simulink model "Lunar_Rocker_N_Arm95_unity"  (R2023b)
settings: Solver=VariableStepAuto  StartTime=0.0  StopTime=160  RelTol=1e-3
libraries: dspnetwork x8, sldrtlib x1
settings Model: Creator=dr  LastModifiedBy=jeric
settings DebuggingCC: UnconnectedInputMsg=warning  UnconnectedOutputMsg=warning  UnconnectedLineMsg=warning
settings ModelReferenceCC: EnableRefExpFcnMdlSchedulingChecks=on
settings RTWCC: DLArmComputeVersion=19.05

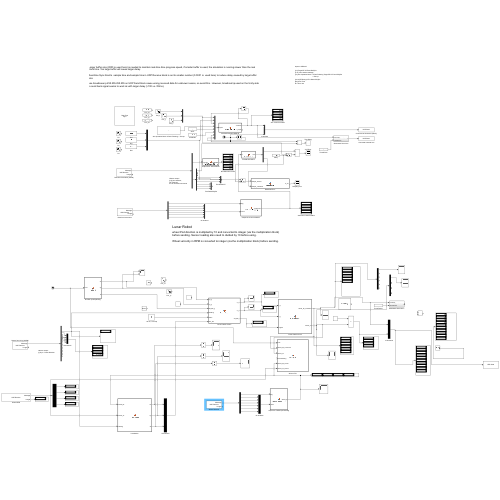
[thumbnail: Simulink's stored preview of the top-level diagram]
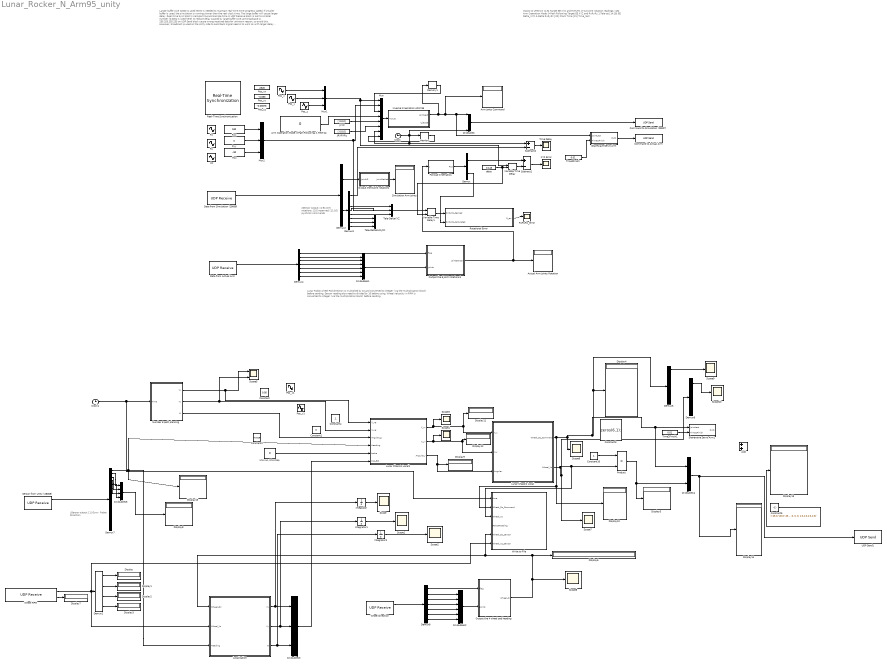
== system Lunar_Rocker_N_Arm95_unity ==
  note: //Sensor output:
      | [1:9] joint rotations;
      | [10] reserved;
      | [11:16] joysticks commands
  note: Larger buffer size {2000 is used here} is needed to maintain real-time time progress speed, if smaller buffer is used, the simulation is running slower than the real clock time. Too large buffer will cause larger delay.
      |
      | Real-time Sync block's sample time and sample time in UDP Receive block is set to smaller number (0.0001 is used here) to reduce delay caused by large buffer size
      |
      | use broadcase ip 255.255.255.255 on UDP Send block cause wrong received data for unknown reason, so avoid this. However, broadcast ip used on the Unity side to send back signal seems to work ok with larger delay (>100 vs <50ms).
  note: Inputs to UR3InvK
      |
      | [1:6] Target EE XYZ and RxRyRz
      | [7:12] Joint rotation readings;
      | [13] Arm Operation Mode: 	0-Path Following Target EE XYZ and RxRyRz
      | 						1:Tele-op
      |
      | [14:19] EE Delta_XYZ & Delta RxRyRz
      | [20] Clock Time
      | [21] Time_last
  note: //Sensor output:
      | [1] Gyro - Robot Direction
  note: Lunar Robot
      |
      | wheel Pod direction is multiplied by 10 and converted to integer (via the multiplication block) before sending. Sensor reading also need to divided by 10 before using.
      |
      | Wheel velcocity in RPM is converted to integer (via the multiplication block) before sending.
  "1 to run, 0 to stop" : Constant  Value=0  OutDataTypeStr=double  SampleTime=0.01
  10 doubles : Mux  Inputs=5
  10 doubles1 : Mux  Inputs=6
  10 doubles2 : Mux  Inputs=6
  10 doubles3 : Mux  Inputs=3
  10 doubles4 : Mux  Inputs=2
  10 doubles5 : Mux
  Actual Arm Joints Rotation : Display
      settings: Decimation=4
  Add : Sum
  Arm Jonts Command : Display
      settings: Decimation=4
  Arm Operation Mode: 0 Path Following; 1 Tele-op : Constant  Value=0
  Clock : Clock
  Clock1 : Clock
  Command to Actual Arm : dspnetwork/UDP Send  remoteURL='192.168.0.226'  remotePort=20001  localURL='0.0.0.0'  localPortSource=Automatically determine  localPort=-1  sendBufferSize=8192  sampletime=-1  blockPlatform=[]  separateLengthPort=0
  Command to Simulation (29007) : dspnetwork/UDP Send  remoteURL='127.0.0.1'  remotePort=29007  localURL='0.0.0.0'  localPortSource=Automatically determine  localPort=-1  sendBufferSize=2500  sampletime=-1  blockPlatform=[]  separateLengthPort=0
  Constant : Constant  Value=0.05  OutDataTypeStr=double  SampleTime=0.1
  Constant1 : Constant  Value=0  OutDataTypeStr=double  SampleTime=0.1
  Constant10 : Constant  OutDataTypeStr=int16
  Constant2 : Constant  Value=-0.628  OutDataTypeStr=double  SampleTime=0.01
  Constant3 : Constant  Value=zeros(6,1);  OutDataTypeStr=int16
  Constant4 : Constant  Value=.1  OutDataTypeStr=double  SampleTime=0.1
  Constant5 : Constant  Value=[-45.0,-45.0,-45.0,-45.0, 0, 0, 1.0,1.0,1.0,1.0]'  OutDataTypeStr=double  SampleTime=0.1
  Data from Actual Arm : dspnetwork/UDP Receive  localURL='0.0.0.0'  localPort=20001  remoteURL='0.0.0.0'  remotePort=-1  recvBufferSize=8192  dims=7  signalDatatype=int16  isComplex=off  isVarSize=off  showBlockingTime=off  blockingTime=0  sampletime=0.0001  blockPlatform=[]
  Data from Simulation (29008) : dspnetwork/UDP Receive  localURL='0.0.0.0'  localPort=29008  remoteURL='127.0.0.1'  remotePort=-1  recvBufferSize=2500  dims=18  signalDatatype=double  isComplex=off  isVarSize=off  showBlockingTime=off  blockingTime=0  sampletime=0.0001  blockPlatform=[]
  Demux : Demux  Outputs=2
  Demux1 : Demux
  Demux2 : Demux  Outputs=2
  Demux3 : Demux  Outputs=9
  Demux4 : Demux  Outputs=7
  Demux5 : Demux  Outputs=6
  Demux6 : Demux
  Demux7 : Demux  Outputs=18
  Demux8 : Demux  Outputs=7
  Display{,1..15} (16 alike) : Display
      Display10 settings: Decimation=4
      Display11 settings: Decimation=4
      Display12 settings: Decimation=4
      Display13 settings: Decimation=4
      Display14 settings: Decimation=4
      Display15 settings: Decimation=4
      Display4 settings: Decimation=6
      Display5 settings: Decimation=4
      Display8 settings: Decimation=4
      Display9 settings: Decimation=4
  Forwad Kinematics : MATLAB Function  TreatAsAtomicUnit=on
  Integrator : Integrator
  Integrator1 : Integrator
  Integrator2 : Integrator
  Inverse Kinematics ARM 95 : MATLAB Function  TreatAsAtomicUnit=on  SystemSampleTime=0.01
  JRXRYRz : Constant  Value=[ 0,0,0]
  JXYZ : Constant  Value=[ 0,0,0]
  Localization : MATLAB Function  TreatAsAtomicUnit=on
  Lunar Chassis Local : MATLAB Function  TreatAsAtomicUnit=on
  Lunar Chassis Local1 : MATLAB Function  TreatAsAtomicUnit=on
  Memory : Memory  InheritSampleTime=on
  Memory1 : Memory  InitialCondition=[0,45,-75,120,90,0]'  InheritSampleTime=on  LinearizeMemory=on  LinearizeAsDelay=on
  Mux : Mux  Inputs=8
  Mux1 : Mux  Inputs=3
  Mux2 : Mux  Inputs=3
  Number 8 path planning : MATLAB Function  TreatAsAtomicUnit=on
  Output the 4 wheel pod heading : MATLAB Function  TreatAsAtomicUnit=on
  Output the 6 Joint rotations : MATLAB Function  TreatAsAtomicUnit=on
  Output the 6 Joint rotations1 : MATLAB Function  TreatAsAtomicUnit=on
  Pos_x : Sin  Amplitude=0.075  Bias=.2595  Frequency=1.57  Phase=1.57  SampleTime=0.01
  Pos_x1 : Sin  Amplitude=.05  Frequency=0.157  SampleTime=0.01
  Pos_xx : Constant  Value=.2345
  Pos_y : Sin  Amplitude=0.15  Bias=-0.053  Frequency=1.57  SampleTime=0.01
  Pos_y1 : Sin  Amplitude=.05  Frequency=0.157  Phase=1.57  SampleTime=0.01
  Pos_yy : Constant  Value=-0.053
  Pos_z : Sin  Amplitude=0.03  Bias=-0.03676  Frequency=6.28  SampleTime=0.01
  Pos_zz : Constant  Value=-0.03676
  Product : Product  OutDataTypeStr=double
  Real-Time Synchronization : sldrtlib/Real-Time Synchronization  SampleTime=0.01  MaxMissedTicks=10000000  ShowMissedTicks=off  YieldWhenWaiting=on
  Rotational Error : MATLAB Function  TreatAsAtomicUnit=on
  Rx : Sin  Amplitude=45  Frequency=.628  SampleTime=0.01
  RxRyRz_Error : Scope
  Rxx : Constant  Value=180
  Ry : Sin  Amplitude=45  Frequency=0.785  SampleTime=0.01
  Ryy : Constant  Value=0
  Rz : Sin  Amplitude=90  Bias=-90  Frequency=0.785  SampleTime=0.01
  Rzz : Constant  Value=-90
  Scope{,1..4,6..10} (10 alike) : Scope
  Scope5 : Scope  NumInputPorts=2
  Sensor from Unity (28008) : dspnetwork/UDP Receive  localURL='0.0.0.0'  localPort=28008  remoteURL='127.0.0.1'  remotePort=-1  recvBufferSize=2500  dims=18  signalDatatype=double  isComplex=off  isVarSize=off  showBlockingTime=off  blockingTime=0  sampletime=0.0001  blockPlatform=[]
  Sharewave Servo Arm : Subsystem
  Sharewave Servo Arm1 : Subsystem
  Simulation Arm Joints : Display
      settings: Decimation=4
  Subtract1 : Sum  Inputs=+-
  Subtract2 : Sum  Inputs=+-
  Tele-DeltaRxRyRz : Mux  Inputs=3
  Tele-DeltaXYZ : Mux  Inputs=3
  Time Delay : Scope
  Time2Finish : Constant  Value=0.01
  Time2Finish1 : Constant  Value=0.01
  UDP Send1 : dspnetwork/UDP Send  remoteURL='127.0.0.1'  remotePort=28007  localURL='0.0.0.0'  localPortSource=Automatically determine  localPort=-1  sendBufferSize=8192  sampletime=-1  blockPlatform=[]  separateLengthPort=0
  Variable Time Delay : VariableTransportDelay  MaximumDelay=10  ZeroDelay=on
  Variable Time Delay1 : VariableTransportDelay  MaximumDelay=10  ZeroDelay=on
  Wheel Direction : dspnetwork/UDP Receive  localURL='0.0.0.0'  localPort=20004  remoteURL='0.0.0.0'  remotePort=-1  recvBufferSize=8192  dims=7  signalDatatype=int16  isComplex=off  isVarSize=off  showBlockingTime=off  blockingTime=0  sampletime=0.0001  blockPlatform=[]
  Wheel RPM : dspnetwork/UDP Receive  localURL='0.0.0.0'  localPort=20002  remoteURL='0.0.0.0'  remotePort=-1  recvBufferSize=8192  dims=4  signalDatatype=int16  isComplex=off  isVarSize=off  showBlockingTime=off  blockingTime=0  sampletime=0.0001  blockPlatform=[]
  Write to File : MATLAB Function  TreatAsAtomicUnit=on
  XYZ Error : Scope
  delay : Constant  Value=0.145
  wires:
  Mux/1 -> Inverse Kinematics ARM 95/1(Inputs)
  Data from Simulation (29008)/1 -> Demux2/1
  Inverse Kinematics ARM 95/1(JointLast) -> Arm Jonts Command/1, Sharewave Servo Arm/1(JointLast), 10 doubles/1, Memory1/1
  Demux/2 -> Rotational Error/2(RxRyRz_calculated)
  Demux/1 -> Subtract1/1
  Subtract1/1 -> XYZ Error/1
  Mux2/1 -> Variable Time Delay1/1, Mux/2
  Forwad Kinematics/1(Pos) -> Demux/1
  Clock/1 -> 10 doubles/5, Mux/7, Subtract2/1, Memory/1
  Memory/1 -> Mux/8
  Mux1/1 -> Variable Time Delay/1, Mux/1
  Demux2/2 -> Demux3/1
  Arm Operation Mode: 0 Path Following; 1 Tele-op/1 -> Mux/4
  Subtract2/1 -> Time Delay/1
  Demux3/1 -> Subtract2/2
  JXYZ/1 -> Mux/5
  JRXRYRz/1 -> Mux/6
  Rotational Error/1(R_err) -> RxRyRz_Error/1
  Sharewave Servo Arm/1(Out1) -> Command to Actual Arm/1
  Time2Finish/1 -> Sharewave Servo Arm/2(Time2Finish)
  Variable Time Delay/1 -> Subtract1/2
  Rxx/1 -> Mux2/1
  Ryy/1 -> Mux2/2
  Rzz/1 -> Mux2/3
  Demux4/4 -> 10 doubles1/3
  Output the 6 Joint rotations1/1(JointSensor) -> Forwad Kinematics/1(J), Actual Arm Joints Rotation/1
  Demux4/3 -> 10 doubles1/2
  Demux4/2 -> 10 doubles1/1
  10 doubles1/1 -> Output the 6 Joint rotations1/2(Joints)
  Demux4/6 -> 10 doubles1/5
  Demux4/1 -> Output the 6 Joint rotations1/1(flag)
  Data from Actual Arm/1 -> Demux4/1
  Demux4/7 -> 10 doubles1/6
  Demux4/5 -> 10 doubles1/4
  Memory1/1 -> Mux/3
  delay/1 -> Variable Time Delay1/2, Variable Time Delay/2
  Variable Time Delay1/1 -> Rotational Error/1(RxRyRz_desired)
  Pos_x/1 -> Mux1/1
  Pos_y/1 -> Mux1/2
  Pos_z/1 -> Mux1/3
  Demux2/1 -> Output the 6 Joint rotations/1(JointVR)
  Output the 6 Joint rotations/1(JointMatlab) -> Simulation Arm Joints/1
  Demux3/8 -> Tele-DeltaRxRyRz/2
  Demux3/9 -> Tele-DeltaRxRyRz/3
  Demux3/6 -> Tele-DeltaXYZ/3
  Demux3/5 -> Tele-DeltaXYZ/2
  Demux3/7 -> Tele-DeltaRxRyRz/1
  Demux3/4 -> Tele-DeltaXYZ/1
  Demux8/5 -> 10 doubles2/4
  Number 8 path planning/2(Vy) -> Lunar Chassis Local1/2(V_yg), Scope5/2
  10 doubles4/1 -> UDP Send1/1, Display14/1
  Wheel RPM/1 -> Localization/2(Wheel_Vs), Write to File/6(Wheel_Vs_Sensor), Demux1/1
  Sensor from Unity (28008)/1 -> Demux7/1
  Lunar Chassis Local/2(Wheel_Vs) -> Write to File/3(Wheel_Vs), Product/2, Scope7/1, Demux6/1
  Demux8/6 -> 10 doubles2/5
  Demux1/3 -> Display2/1
  Demux1/4 -> Display3/1
  Localization/3(W) -> Integrator2/1, 10 doubles3/3
  Localization/2(Vy) -> Integrator1/1, 10 doubles3/2
  Integrator/1 -> Scope/1
  Constant5/1 -> Display13/1
  Demux6/1 -> Scope10/1
  Constant10/1 -> Product/1
  Demux8/2 -> 10 doubles2/1
  Lunar Chassis Local1/2(V_yr) -> Display12/1, Lunar Chassis Local/2(V_y), Scope4/1
  Wheel RPM/2 -> Display7/1
  Demux5/1 -> Scope9/1
  Integrator2/1 -> Scope2/1
  10 doubles5/1 -> Display8/1
  Demux7/2 -> 10 doubles5/1
  "1 to run, 0 to stop"/1 -> Lunar Chassis Local1/5(brake)
  Lunar Chassis Local/1(Wheel_Ds_Command) -> Display10/1, Write to File/2(Wheel_Ds_Command), 10 doubles4/1, Sharewave Servo Arm1/1(JointLast), Demux5/1, Display4/1, Scope6/1
  Output the 4 wheel pod heading/1(Wheel_D) -> Write to File/5(Wheel_Ds_sensor), Localization/1(Wheel_Ds), Display6/1, Scope8/1
  Demux7/3 -> 10 doubles5/2
  Demux8/7 -> 10 doubles2/6
  Demux7/1 -> Localization/3(Heading), Display15/1, Lunar Chassis Local1/4(Heading)
  Demux8/3 -> 10 doubles2/2
  Demux1/2 -> Display1/1
  10 doubles2/1 -> Output the 4 wheel pod heading/2(Joints)
  Demux8/4 -> 10 doubles2/3
  Lunar Chassis Local1/3(Angular_r) -> Display9/1, Lunar Chassis Local/3(Angular)
  Localization/1(Vx) -> Integrator/1, 10 doubles3/1
  Demux7/4 -> 10 doubles5/3
  Integrator1/1 -> Scope1/1
  Number 8 path planning/1(Vx) -> Lunar Chassis Local1/1(V_xg), Scope5/1
  Product/1 -> 10 doubles4/2, Display5/1
  Number 8 path planning/3(W) -> Lunar Chassis Local1/3(Angular_g)
  Demux8/1 -> Output the 4 wheel pod heading/1(flag)
  Lunar Chassis Local1/1(V_xr) -> Scope3/1, Display11/1, Lunar Chassis Local/1(V_x)
  Wheel Direction/1 -> Demux8/1
  Demux7/5 -> 10 doubles5/4
  10 doubles3/1 -> Lunar Chassis Local1/6(Pos_Est)
  Time2Finish1/1 -> Sharewave Servo Arm1/2(Time2Finish)
  Demux1/1 -> Display/1
  10 doubles/1 -> Command to Simulation (29007)/1
  Clock1/1 -> Write to File/1(time), Number 8 path planning/1(Time)

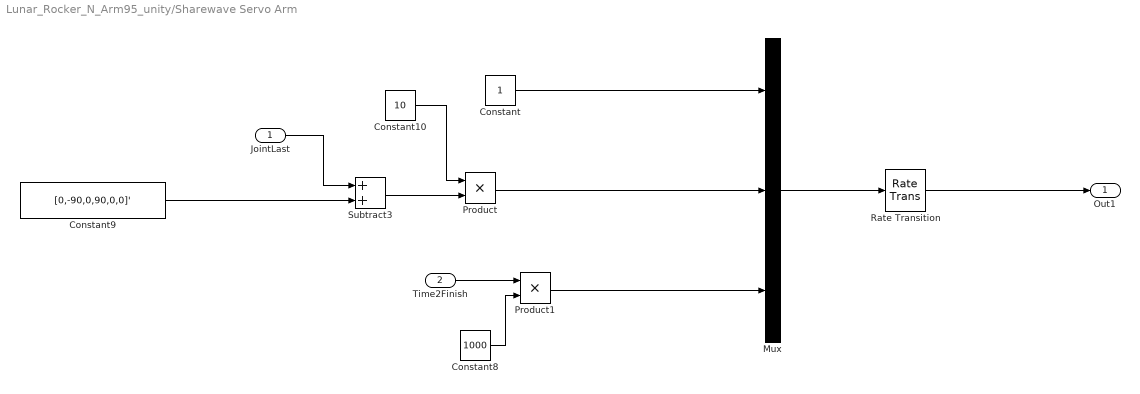
== system Lunar_Rocker_N_Arm95_unity/Sharewave Servo Arm ==
  JointLast : Inport
  Time2Finish : Inport  Port=2
  Constant : Constant  OutDataTypeStr=int16  SampleTime=0.1
  Constant10 : Constant  Value=10  OutDataTypeStr=int16
  Constant8 : Constant  Value=1000  OutDataTypeStr=int16
  Constant9 : Constant  Value=[0,-90,0,90,0,0]'  OutDataTypeStr=int16
  Mux : Mux  Inputs=3
  Product : Product  OutDataTypeStr=int16
  Product1 : Product  OutDataTypeStr=int16
  Rate Transition : RateTransition  OutPortSampleTime=0.01
  Subtract3 : Sum  OutDataTypeStr=int16
  Out1 : Outport
  wires:
  JointLast/1 -> Subtract3/1
  Mux/1 -> Rate Transition/1
  Constant/1 -> Mux/1
  Constant8/1 -> Product1/2
  Constant9/1 -> Subtract3/2
  Constant10/1 -> Product/1
  Subtract3/1 -> Product/2
  Rate Transition/1 -> Out1/1
  Product/1 -> Mux/2
  Time2Finish/1 -> Product1/1
  Product1/1 -> Mux/3

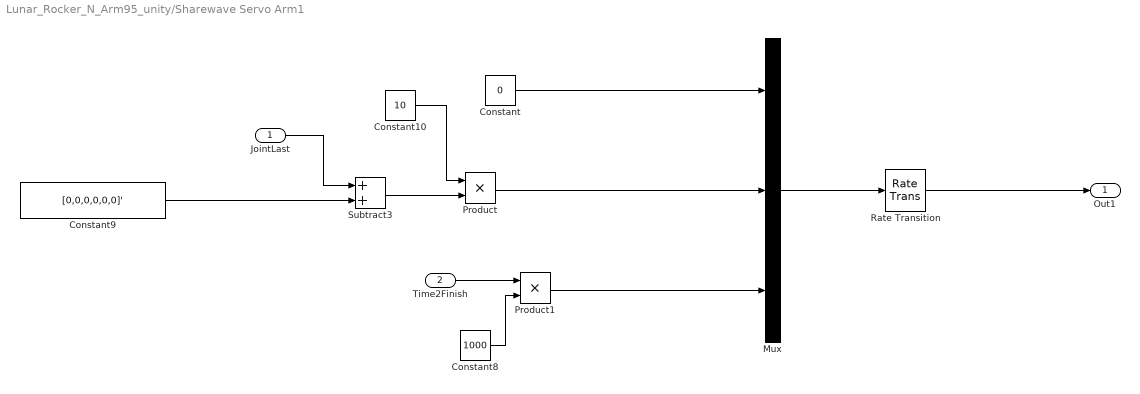
== system Lunar_Rocker_N_Arm95_unity/Sharewave Servo Arm1 ==
  JointLast : Inport
  Time2Finish : Inport  Port=2
  Constant : Constant  Value=0  OutDataTypeStr=int16  SampleTime=0.1
  Constant10 : Constant  Value=10  OutDataTypeStr=int16
  Constant8 : Constant  Value=1000  OutDataTypeStr=int16
  Constant9 : Constant  Value=[0,0,0,0,0,0]'  OutDataTypeStr=int16
  Mux : Mux  Inputs=3
  Product : Product  OutDataTypeStr=int16
  Product1 : Product  OutDataTypeStr=int16
  Rate Transition : RateTransition  OutPortSampleTime=0.01
  Subtract3 : Sum  OutDataTypeStr=int16
  Out1 : Outport
  wires:
  JointLast/1 -> Subtract3/1
  Mux/1 -> Rate Transition/1
  Constant/1 -> Mux/1
  Constant8/1 -> Product1/2
  Constant9/1 -> Subtract3/2
  Constant10/1 -> Product/1
  Subtract3/1 -> Product/2
  Rate Transition/1 -> Out1/1
  Product/1 -> Mux/2
  Time2Finish/1 -> Product1/1
  Product1/1 -> Mux/3

== matlab function Lunar_Rocker_N_Arm95_unity/Write to File ==
  settings: updateMethod=DISCRETE
  data: time input; Wheel_Ds_Command input; Wheel_Vs input; RobotHeading input; Wheel_Ds_sensor input; Wheel_Vs_Sensor input
function  WriteToFile(time, Wheel_Ds_Command, Wheel_Vs, RobotHeading, Wheel_Ds_sensor, Wheel_Vs_Sensor)
persistent  fileID; 

if isempty(fileID)
    fileID = fopen('log.txt','w');
    fprintf(fileID,'%6s %6s %6s %6s %6s %6s %6s %6s %6s','Time','D1','D2','D3','D4', 'V1','V2','V3','V4');
    fprintf(fileID,'%6s %6s %6s %6s %6s %6s %6s %6s %6s','Angle','D1_s','D2_s','D3_s','D4_s', 'V1_s','V2_s','V3_s','V4_s');
    fprintf(fileID,' \r\n');
end


fprintf(fileID,'%6.2f %6.1f %6.1f %6.1f %6.1f %6.1f %6.1f %6.1f %6.1f', time, Wheel_Ds_Command(1), Wheel_Ds_Command(2), Wheel_Ds_Command(3), Wheel_Ds_Command(4), Wheel_Vs(1), Wheel_Vs(2), Wheel_Vs(3), Wheel_Vs(4));
fprintf(fileID,'%6.1f %6.1f %6.1f %6.1f %6.1f %6d %6d %6d %6d', RobotHeading, Wheel_Ds_sensor(1), Wheel_Ds_sensor(2), Wheel_Ds_sensor(3), Wheel_Ds_sensor(4), Wheel_Vs_Sensor(1), Wheel_Vs_Sensor(2), Wheel_Vs_Sensor(3), Wheel_Vs_Sensor(4));
fprintf(fileID,' \r\n');

== matlab function Lunar_Rocker_N_Arm95_unity/Output the 6 Joint rotations ==
  data: JointVR input; JointMatlab output
function JointMatlab  = MatlabMaping6Joints(JointVR)
JointMatlab  = zeros (6,1);
JointMatlab(1:6) = JointVR(1:6);

== matlab function Lunar_Rocker_N_Arm95_unity/Forwad Kinematics ==
  data: J input; Pos output
function Pos  = LunarArmFK(J)
%UR3 robot arm

%cal Jacobian using 5.1.27, page 115, Robot Dyn and Control by Spong
Joint = zeros(6,1);
Pos = zeros(6,1);

Degree2Radian = pi/180;
 


%initial joint position
Joint(1)= J(1)*Degree2Radian;
Joint(2)= J(2)*Degree2Radian;
Joint(3)= J(3)*Degree2Radian;
Joint(4)= J(4)*Degree2Radian;
Joint(5)= J(5)*Degree2Radian;
Joint(6)= J(6)*Degree2Radian;
  

PTool=[0;0;0;1]; %The Tool or tip position expressed wrt the last frame physical dimension



dh = [   0              0           0           Joint(1); 
             pi/2           0           0           Joint(2);
             0              0.175       0           Joint(3);
             0              0.155        0.053           Joint(4);
             pi/2            0           0.0765     Joint(5);
             -pi/2           0           0.083     Joint(6)];

 
T=[1 0 0 0;0 1 0 0; 0 0 1 0; 0 0 0 1]; %INITIAL  Transformation matrix

for m=1:6
T=T*[cos(dh(m,4))                    -sin(dh(m,4))                0               dh(m,2)
    sin(dh(m,4))*cos(dh(m,1))   cos(dh(m,4))*cos(dh(m,1))   -sin(dh(m,1))       -sin(dh(m,1))*dh(m,3)
    sin(dh(m,4))*sin(dh(m,1))   cos(dh(m,4))*sin(dh(m,1))   cos(dh(m,1))       cos(dh(m,1))*dh(m,3)
    0                               0                           0               1];
%Axis(1:3,m)=T(1:3,3);
%Origin(1:3,m)= T(1:3,4);
end

PEndTemp=T*PTool;

Pos(1:3)= PEndTemp(1:3);
%[AXInitial,AYInitial,AZInitial] based on Fixed Angle
 

[Pos(4) Pos(5) Pos(6)]= R2FixAngle(T(1:3,1:3));
Pos(4:6) = Pos(4:6)/Degree2Radian;

function [AX,AY,AZ]= R2FixAngle(R) 

MINA=0.0001; %minimun we consider to be 0 degree

AY= atan2(-R(3,1), sqrt(R(1,1)^2+R(2,1)^2));

CAY=cos(AY);

if abs(CAY)>MINA
    AZ=atan2(R(2,1)/CAY, R(1,1)/CAY);
    AX=atan2(R(3,2)/CAY, R(3,3)/CAY);
elseif AY>0 % AY=90 degree
   AY=pi/2;
   AZ=0; %this is a convention to choose AZ to be zero, see page 47
   AX=atan2(R(1,2), R(2,2));
else  % AY=-90 degree
   AY=-pi/2;
   AZ=0; %this is a convention to choose AZ to be zero, see page 47
   AX=-atan2(R(1,2), R(2,2));
end

== matlab function Lunar_Rocker_N_Arm95_unity/Rotational Error ==
  data: RxRyRz_desired input; R_err output; RxRyRz_calculated input
function R_err  = RotationErr(RxRyRz_desired, RxRyRz_calculated)

R1 = zeros(3,3);
R2 = zeros(3,3);
Rerror = zeros(3,3);

Degree2Radian = pi/180;
 
R1= FixAngle2R(RxRyRz_desired*Degree2Radian);
R2= FixAngle2R(RxRyRz_calculated*Degree2Radian);




Rerror = R1*(R2');
R_err = 0.5*[Rerror(3,2)-Rerror(2,3); Rerror(1,3)-Rerror(3,1);Rerror(2,1)-Rerror(1,2)];


%Fixed Angle representation page 45, intro to robotics
%Definition: Describing the orientation of frame B is as follows:
%start  with the frame coincident with a known reference frame A. First
%rotate B about axis XA by an angle AngleX, then rotate about YA by an
%angle AngleY, and then rotate about ZA by an angle AngleZ.

function [R]= FixAngle2R(AngleXYZ) 

cX  = cos (AngleXYZ(1));
sX  =   sin(AngleXYZ(1));
cY  =   cos (AngleXYZ(2));
sY  =   sin(AngleXYZ(2));
cZ  =   cos (AngleXYZ(3));
sZ  =   sin(AngleXYZ(3));

R=[cZ*cY cZ*sY*sX-sZ*cX cZ*sY*cX+sZ*sX;
   sZ*cY sZ*sY*sX+cZ*cX sZ*sY*cX-cZ*sX;
   -sY  cY*sX   cY*cX];

== matlab function Lunar_Rocker_N_Arm95_unity/Inverse Kinematics ARM 95 ==
  data: Inputs input; JointLast output; t_lapse output
function [JointLast, t_lapse]  = LunarArmInvK (Inputs)
persistent  PositionLast  RotationLast;

if isempty(PositionLast)
    PositionLast =zeros(3,1);
end

if isempty(RotationLast)
    RotationLast =zeros(3,1);
end

 
t_lapse = Inputs(20)- Inputs(21);

if Inputs(20) > 0.0 % delay start to make sure sensor data from the VR robot has arrived, during delay, send out the initial joint position 
 
% LEFT  ARM
% This function will generate the joint angle set for each joint on left
% arm based on drawing a circle on XZ plane, radius is RD.
% there are many import parameters is based on physical arm dimensions.
% please contact Dr Robot Inc for further information.

% The demo code is just for 'demo' use.

%cal Jacobian using 5.1.27, page 115, Robot Dyn and Control by Spong
%JInit

steps=5; 

Joint = zeros(6,steps+1);
JointWS = zeros(6,2);
Origin = zeros(3,6);
Axis = zeros(3,6);
PEnd = zeros (3,steps);
Jaco = zeros (6,6);
PTarget = zeros(3, steps+1);
FATarget = zeros(3, steps+1);
ODelta = zeros(3,steps);
WJointLtd = zeros (6,6);
JointLast = zeros (6,1);
RTeleDelta = eye(3,3);
finalPos = zeros(3,1);
finalRxRyRz = zeros(3,1);
PTeleDelta = zeros (3,1);  
Degree2Radian = pi/180;
RxRyRzTeleDelta = zeros(3,1);
RJ5 = zeros(3,3);

%initial joint position
Joint(1,1)= Inputs(7)*Degree2Radian;
Joint(2,1)= Inputs(8)*Degree2Radian;
Joint(3,1)= Inputs(9)*Degree2Radian;
Joint(4,1)= Inputs(10)*Degree2Radian;
Joint(5,1)= Inputs(11)*Degree2Radian;
Joint(6,1)= Inputs(12)*Degree2Radian;

%########################physical dimensions #############################
%Joint limit in degrees
JointLtd=[  -360,   360;
             -360,   360;
            -360,   360;
            -360,   360;
            -360,   360;
            -9000,   9000];
JointLtdExRate = 50; %Joint ltd avoidance exp increase rate, if this rate is too small, e.g. 10 or 1, it may exceed the limit a bit; 
JointSB=20; % safe zone before reaching joint limit, joint limit avoidance scheme starts action when entering the safe zone. effect grows exponentially
%Convert the safe operation zone (with a boundary of JointSB before the
%limit) from degree into the RAD
for i=1:6
           JointWS(i,1)=(JointLtd(i,1)+JointSB)*Degree2Radian;
           JointWS(i,2)=(JointLtd(i,2)-JointSB)*Degree2Radian;
end
       
T=[1 0 0 0;0 1 0 0; 0 0 1 0; 0 0 0 1]; %INITIAL  Transformation matrix
PTool=[0;0;0;1]; %The Tool or tip position expressed wrt the last frame physical dimension
%Catisian space task weighting, i.e. position and orientation tracking task
%weight, smaller , less significant to track, i.e. by setting WEnd(4,4)
%smaller (e.g. 0.01 while others are 1), the rotation along RX axis will not be tracked precisely.
%!!!!!!!!!!!!!!!!!!!!CHANGE HERE

WEnd=[1 0 0 0 0 0;
    0 1 0 0 0 0;
    0 0 1 0 0 0;
    0 0 0 .01 0 0;
    0 0 0 0 .01 0;
    0 0 0 0 0 .01];           %0.01

%Joint space weighting matrix, larger number will reduce the joint motion,
%i.e. the unit WJoint(6,6)=100, while others are "1" then the joint 6 will
%move very little.
%!!!!!!!!!!!!!!!!!!!!CHANGE HERE
WJoint=[1 0 0 0 0 0;
        0 1 0 0 0 0;
        0 0 1 0 0 0;
        0 0 0 .1 0 0;
        0 0 0 0 .1 0;
        0 0 0 0 0 .1];

 
DF2= 0.05; %0.15; %.015; %Damping factor square, larger, slower tracking, bigger tracking error, but more robust to singularity 


for k = 1:steps

    dh = [   0              0           0           Joint(1,k); 
             pi/2           0           0           Joint(2,k);
             0              0.175       0           Joint(3,k);
             0              0.155       0.053           Joint(4,k);
             pi/2            0           0.0765     Joint(5,k);
             -pi/2           0           0.083     Joint(6,k)];
 
T=[1 0 0 0;0 1 0 0; 0 0 1 0; 0 0 0 1]; %INITIAL  Transformation matrix

for m=1:6
T=T*[cos(dh(m,4))                    -sin(dh(m,4))                0               dh(m,2)
    sin(dh(m,4))*cos(dh(m,1))   cos(dh(m,4))*cos(dh(m,1))   -sin(dh(m,1))       -sin(dh(m,1))*dh(m,3)
    sin(dh(m,4))*sin(dh(m,1))   cos(dh(m,4))*sin(dh(m,1))   cos(dh(m,1))       cos(dh(m,1))*dh(m,3)
    0                               0                           0               1];
Axis(1:3,m)=T(1:3,3);
Origin(1:3,m)= T(1:3,4);
%if m==5 % copy the second last joint, (before the hand) Rotation
%    RJ5 = T(1:3,1:3);
%end

end

PEndTemp=T*PTool;
PEnd(1:3,k)=PEndTemp(1:3); %tip position in origin frame

%Jacobian upper part , i.e. the linear velocity part
Jaco(1:3,1)= cross (Axis (1:3,1), (PEnd (1:3,k) - Origin(1:3,1)));
Jaco(1:3,2)= cross (Axis (1:3,2), (PEnd (1:3,k)- Origin(1:3,2)));
Jaco(1:3,3)= cross (Axis (1:3,3), (PEnd (1:3,k)- Origin(1:3,3)));
Jaco(1:3,4)= cross (Axis (1:3,4), (PEnd (1:3,k)- Origin(1:3,4)));
Jaco(1:3,5)= cross (Axis (1:3,5), (PEnd (1:3,k)- Origin(1:3,5)));
Jaco(1:3,6)= cross (Axis (1:3,6), (PEnd (1:3,k)- Origin(1:3,6)));

%Jacobian lower part , i.e. the angular velocity part
Jaco(4:6,1)= Axis (1:3,1);
Jaco(4:6,2)= Axis (1:3,2);
Jaco(4:6,3)= Axis (1:3,3);
Jaco(4:6,4)= Axis (1:3,4);
Jaco(4:6,5)= Axis (1:3,5);
Jaco(4:6,6)= Axis (1:3,6);

if k==1 %cal the initial posotition and orientation from the initial joint reading
%target position, should use the sensor reading to calculate the X,Y,Z and
%plan the end effector motion accordingly to avoid rapid movement at start

PInitial    = PEnd(1:3,1);
RInitial    = T(1:3,1:3);
    
%Initialize the tip motion Target 
PTarget(1, 1) = PInitial(1);
PTarget(2, 1) = PInitial(2);
PTarget(3, 1) = PInitial(3) ;

InitialRxRyRZ=R2FixAngle(RInitial);
 
FATarget(1:3,1) = InitialRxRyRZ; %using Fixed-Angle representation page 47, intro to robotics

% set the final target position and RxRyRz
    if Inputs(13) >=1 % 1: tele-operation on end-effector, using Mode switching Initial pos + delat pos as the final target 
        magPosCommand = norm(Inputs(14:16));
        magRotCommand = norm(Inputs(17:19)); 

     if magPosCommand < 0.2  %no motion needed
         PTeleDelta = zeros(3,1);
     else
         PTeleDelta =RInitial*Inputs(14:16)*t_lapse*0.1;
     end

     if magRotCommand < 0.2 %no rotation needed
        RTeleDelta = eye(3,3);
     else
        RxRyRzTeleDelta = Inputs(17:19)*t_lapse*0.5;
        RTeleDelta = FixAngle2R (RxRyRzTeleDelta(1:3));   
     end
        
        finalPos = PositionLast + PTeleDelta;
        finalRxRyRz=R2FixAngle(FixAngle2R(RotationLast*Degree2Radian)*RTeleDelta)*180/pi;
        %finalRxRyRz = Inputs (4:6);
     
    else % =0 path following
        finalPos = Inputs (1:3);
        finalRxRyRz = Inputs (4:6);
    end
end    


%linear planning 
PTarget(1, k+1) = PTarget(1,1) + (finalPos(1)-PTarget(1,1))/steps*k;
PTarget(2, k+1) = PTarget(2,1) + (finalPos(2)-PTarget(2,1))/steps*k ;
PTarget(3, k+1) = PTarget(3,1) + (finalPos(3)-PTarget(3,1))/steps*k;
%PTarget(3, k+1) = PTarget(3,1) - RD - RD*cos(pi+ 2*pi*k/steps);


%planning the orientation motion

FATarget(1,k+1)= finalRxRyRz(1)*Degree2Radian ; 
FATarget(2,k+1)= finalRxRyRz(2)*Degree2Radian ;
FATarget(3,k+1)= finalRxRyRz(3)*Degree2Radian ;

RTarget = FixAngle2R(FATarget(1:3,k+1));

%tip motion delta
PDelta= PTarget(1:3,k+1)-PEnd(1:3,k);
%Rotation error
Rerror = RTarget*(T(1:3,1:3)');
ODelta(1:3,k) = 0.5*[Rerror(3,2)-Rerror(2,3); Rerror(1,3)-Rerror(3,1);Rerror(2,1)-Rerror(1,2)];

%Least square pseudo inverse of J
JacoP=Jaco(1:6,1:6);
%Jw=transpose(JacoP)*inv(JacoP*transpose(JacoP)+ DF2*eye(6));


%Joint limit avoidance
for i=1:6
    if Joint(i,k)>JointWS(i,2)
        JointOver= Joint(i,k)-JointWS(i,2);
    elseif     Joint(i,k) <JointWS(i,1)
        JointOver= JointWS(i,1)-Joint(i,k) ;
    else
       JointOver=0;     
   end   
WJointLtd(i,i)=WJoint(i,i)*exp(JointLtdExRate*JointOver); %Augment the WJoint weighting matrix with the Joint Limit Avoidance, closer to the limit, the Weighting unit will increase exponentially, and leading to smaller velocity till stop, therefore avoiding exceeding the limit
end

Jw=inv(transpose(JacoP)*WEnd*JacoP+ DF2*(WJointLtd))*transpose(JacoP)*WEnd;

%conJ=cond(JacoP)
%Jw=inv(Jaco);
%inverse kinematic of delta joint motion 

JDelta= Jw*[PDelta;ODelta(1:3,k)]; 

%orientation only
%Jw=W1*transpose(Jaco(4:6,1:6))*inv(Jaco(4:6,1:6)*W1*transpose(Jaco(4:6,1:6)));
%JDelta= Jw*[ODelta];

%with error on joint trackin
%Joint(1:6,k+2)=Joint(1:6,k+1)+JDelta + dot (JDelta, [0.5*(rand-0.5);0.5*(rand-0.5);0.5*(rand-0.5);0.5*(rand-0.5);0.2*(rand-0.5);0.2*(rand-0.5)]);
%here is what the robot arm controller should do: drive the arm to the
%position we need:
Joint(1:6,k+1)=Joint(1:6,k)+JDelta; 
end


JointLast(1:6) = Joint(1:6,k+1)/Degree2Radian;
PositionLast =  finalPos; %storrage of last pos target command 
RotationLast = finalRxRyRz;

else
    %initial position
    JointLast = [0, 45,-75, 120, 90, 0]';
    PositionLast =[0.3345, -0.053,-0.03676]';
    RotationLast = [180,0,-90]';
end
 

function AxAyAZ= R2FixAngle(R) 

MINA=0.0001; %minimun we consider to be 0 degree

AY= atan2(-R(3,1), sqrt(R(1,1)^2+R(2,1)^2));

CAY=cos(AY);

if abs(CAY)>MINA
    AZ=atan2(R(2,1)/CAY, R(1,1)/CAY);
    AX=atan2(R(3,2)/CAY, R(3,3)/CAY);
elseif AY>0 % AY=90 degree
   AY=pi/2;
   AZ=0; %this is a convention to choose AZ to be zero, see page 47
   AX=atan2(R(1,2), R(2,2));
else  % AY=-90 degree
   AY=-pi/2;
   AZ=0; %this is a convention to choose AZ to be zero, see page 47
   AX=-atan2(R(1,2), R(2,2));
end
AxAyAZ = [AX AY AZ]';

%Fixed Angle representation page 45, intro to robotics
%Definition: Describing the orientation of frame B is as follows:
%start  with the frame coincident with a known reference frame A. First
%rotate B about axis XA by an angle AngleX, then rotate about YA by an
%angle AngleY, and then rotate about ZA by an angle AngleZ.

function [R]= FixAngle2R(AngleXYZ) 

cX  = cos (AngleXYZ(1));
sX  =   sin(AngleXYZ(1));
cY  =   cos (AngleXYZ(2));
sY  =   sin(AngleXYZ(2));
cZ  =   cos (AngleXYZ(3));
sZ  =   sin(AngleXYZ(3));

R=[cZ*cY cZ*sY*sX-sZ*cX cZ*sY*cX+sZ*sX;
   sZ*cY sZ*sY*sX+cZ*cX sZ*sY*cX-cZ*sX;
   -sY  cY*sX   cY*cX];

== matlab function Lunar_Rocker_N_Arm95_unity/Localization ==
  data: Wheel_Ds input; Vx output; Vy output; W output; Wheel_Vs input; Heading input
function [Vx, Vy, W]  = Localization(Wheel_Ds, Wheel_Vs, Heading)

 

V_xr =0;
V_yr=0;
W=0;
PIH = zeros (3,8);
V_wheel = zeros(8,1);
V_robot = zeros(3,1);
 
Wheel_Ds  = double (Wheel_Ds  *pi/180.0);
 
V2RPM = 60.0/ (3.1415926*0.1);  % convert from m/s to RPM
 
Wheel_Vs = double (Wheel_Vs) /V2RPM;

L2 = 0.358/2.0; % half the length
W2 = 0.372/2.0;

H = [   1,  0,    -L2;
        0,  1,    -W2;
        1,  0,    -L2;
        0,  1,    W2;
        1,  0,    L2;
        0,  1,    -W2;
        1,  0,    L2;
        0,  1,    W2;];

PIH = inv(H'*H)*H';

for i =1:4
    V_wheel(2*i-1,1) = -Wheel_Vs(i)*sin(Wheel_Ds(i));
    V_wheel(2*i,1) = Wheel_Vs(i)*cos(Wheel_Ds(i));
end
V_robot = PIH*V_wheel;

V_xr = V_robot(1);
V_yr = V_robot(2);
W = V_robot(3) *180/pi;

%mapping to global frame

Heading = Heading  * 3.14/180;

Vx= (cos (Heading) *V_xr - sin(Heading) *V_yr) ;
Vy= (sin (Heading) *V_xr + cos(Heading) *V_yr) ;

== matlab function Lunar_Rocker_N_Arm95_unity/Output the 6 Joint rotations1 ==
  data: flag input; JointSensor output; Joints input
function JointSensor  = JointSensorMapping(flag, Joints)
persistent  Joints_last;
JointSensor =zeros(6,1);

if isempty(Joints_last)
    Joints_last =zeros(6,1);
end

if (flag == 1) && isempty (Joints) ~= true
    Joints_last = double (Joints)/10 - [0,-90,0,90,0,0]';
end

JointSensor = Joints_last;

== matlab function Lunar_Rocker_N_Arm95_unity/Lunar Chassis Local ==
  settings: updateMethod=DISCRETE
  data: V_x input; V_y input; Wheel_Ds_Command output; Angular input; Wheel_Vs output
function [Wheel_Ds_Command, Wheel_Vs]  = LunarChassis(V_x, V_y , Angular)
%output Wheel velocity in RPM

persistent Wheel_Ds_last Wheel_Ds_NoLimit Wheel_Ds_NoLimit_last ;  

if  isempty (Wheel_Ds_last) 
     Wheel_Ds_last =zeros(6,1);
end
if  isempty (Wheel_Ds_NoLimit) 
     Wheel_Ds_NoLimit = zeros(6,1);
     Wheel_Ds_NoLimit_last = zeros(6,1);
end
if  isempty (Wheel_Ds_NoLimit_last)
     Wheel_Ds_NoLimit_last = zeros(6,1);
end

 


Wheel_Ds= zeros(6,1); % only use the first 4, but the protocol needs a lenght of 6
Wheel_Vs= zeros(4,1);

Radian2Degree = 180/pi;
V2RPM = 60.0/ (3.1415926*0.1);  % convert from m/s to RPM
Length = 0.33472;
Width = 0.35038;

A = V_x + Angular *Length/2;
B = V_x - Angular *Length/2;
C = V_y + Angular *Width/2;

D = V_y - Angular *Width/2;
%LF
Wheel_Vs(1) = sqrt(B*B + D*D)*V2RPM;
Wheel_Ds(1) = -atan2(B,D)*Radian2Degree;
%RF
Wheel_Vs(2) = sqrt(B*B + C*C)*V2RPM;
Wheel_Ds(2) = -atan2(B,C)*Radian2Degree;
%LR
Wheel_Vs(3) = sqrt(A*A + D*D)*V2RPM ;
Wheel_Ds(3) = -atan2(A,D)*Radian2Degree;
%RR
Wheel_Vs(4) = sqrt(A*A + C*C)*V2RPM ;
Wheel_Ds(4) = -atan2(A,C)*Radian2Degree;

% Atan2 will return pi - -pi and may jump from pi to -pi, we need to
% process it, if the turning is over 180, take the direction with less
% truning, make sure turning is always less than 180

for i = 1:4 
    deltaRotation = Wheel_Ds(i) - Wheel_Ds_last(i);
    if (deltaRotation < -180)
        deltaRotation =   deltaRotation + 360;
    end
    if (deltaRotation > 180)
        deltaRotation = deltaRotation - 360;
    end
   
    Wheel_Ds_NoLimit(i) = Wheel_Ds_NoLimit(i)+ deltaRotation;
    Wheel_Ds_last(i)  = Wheel_Ds(i);
end



% since we could reverse the motor power instead turn the motor pod, if the
% turning is over 90 degree, we could reverse the wheel direction.

Wheel_Ds_Command = Wheel_Ds_NoLimit;

for i = 1:4
    if  Wheel_Ds_Command(i) -Wheel_Ds_NoLimit_last(i) > 90  
        Wheel_Ds_Command(i)= Wheel_Ds_Command(i)-180;
        Wheel_Vs(i) = - Wheel_Vs(i) ;
    elseif  Wheel_Ds_Command(i) -Wheel_Ds_NoLimit_last(i) < -90 
        Wheel_Ds_Command(i)= Wheel_Ds_Command(i) + 180;
        Wheel_Vs(i) = - Wheel_Vs(i) ;
    end
    Wheel_Ds_NoLimit_last(i) = Wheel_Ds_Command(i);
end

== matlab function Lunar_Rocker_N_Arm95_unity/Lunar Chassis Local1 ==
  data: V_xg input; V_yg input; V_xr output; Angular_g input; V_yr output; Heading input; Angular_r output; brake input; Pos_Est input
function [V_xr, V_yr, Angular_r]  = GlobaltoLocal(V_xg, V_yg , Angular_g, Heading, brake, Pos_Est)
%mapping global command to robot local frame
Heading = Heading  * 3.14/180;

V_xr =0;
V_yr =0;

% 
% persistent err_x_last err_y_last err_x_int err_y_int
% 
% if isempty(err_y_last)
%     err_x_last =0;
%     err_y_last =0;
%     err_x_int =0;
%     err_y_int =0;
% end
% err_x =0;
% err_y =0;
% % Kp control
% kp = 0;
% kd = 0;
% ki = 0.1;
% 
% 
% err_x = V_xg-Pos_Est(1);
% err_y = V_yg-Pos_Est(2);
% 
% err_x_int = err_x_int + err_x*0.01
% err_y_int = err_y_int + err_y*0.01
% 
% V_xg = V_xg + ki*err_x_int % + kp *err_x + kd*(err_x - err_x_last);
% V_yg = V_yg + ki*err_y_int %+ kp *err_y + kd*(err_y - err_y_last);
% 
% err_x_last = err_x;
% err_y_last = err_y;

V_xr= (cos (Heading) *V_xg + sin(Heading) *V_yg)*brake;
V_yr= (-sin (Heading) *V_xg + cos(Heading) *V_yg)*brake;
Angular_r = Angular_g*brake;

== matlab function Lunar_Rocker_N_Arm95_unity/Number 8 path planning ==
  data: Time input; Vx output; Vy output; W output
function [Vx, Vy, W]  = Path_8 (Time)

Vx=0;
Vy=0;
W=0;
delayStart =2;
Time1 = 25;
Time2 = 25;

W1=2*pi/Time1;
W2=2*pi/Time2;
Time_Total = Time1 + Time2;

r1=2.5;
r2=2.5;


if  Time < delayStart
Vx=0;
Vy=0;
W=0;

elseif Time < delayStart+ Time1
    Vx = -W1*r1*sin(W1*(Time-delayStart)+pi);
    Vy = W1*r1*cos(W1*(Time-delayStart));
    W= pi/Time1;%0; %(pi*pi/Time_Total)*sin(pi/Time_Total *(Time-delayStart));

elseif Time <delayStart + Time1+Time2
    Vx = W2*r2*sin(W2*(Time-Time1-delayStart)+pi);
    Vy = W2*r2*cos(W2*(Time-Time1-delayStart));
    W= pi/Time2; % 0; %(pi*pi/Time_Total)*sin(pi/Time_Total *(Time-delayStart));
else



Vx=0;
Vy=0;
W=0;
end

== matlab function Lunar_Rocker_N_Arm95_unity/Output the 4 wheel pod heading ==
  data: flag input; Wheel_D output; Joints input
function Wheel_D  = JointSensorMapping(flag, Joints)
persistent  Joints_last;
 

if isempty(Joints_last)
     Joints_last = [0, 0,0,0,0,0]';
  
end

if isempty (Joints) ~= true
    Joints_last = double (Joints)/10;
end

Wheel_D = Joints_last (1:4);
